simulink model "lab1_model"  (R2018a)
settings: Solver=VariableStepAuto  StartTime=0.0  StopTime=8  RelTol=1e-3
values from neighbouring files (symbols this model uses):
  Jtot = 7.226    [Lab1_script.m]
  Kb = 2    [Lab1_script.m]
  KCS = 0.5    [Lab1_script.m]
  Kf = 0.1    [Lab1_script.m]
  KSS = 0.0433    [Lab1_script.m]
  ntotKt = 1.8    [Lab1_script.m]
  r_itot = 0.0615    [Lab1_script.m]
  Ra = 1    [Lab1_script.m]
  RocwAvor_itot = 0.6154    [Lab1_script.m]
libraries: simulink x3
settings Model: Creator=Mohamed Badr  LastModifiedBy=Mohamed Badr

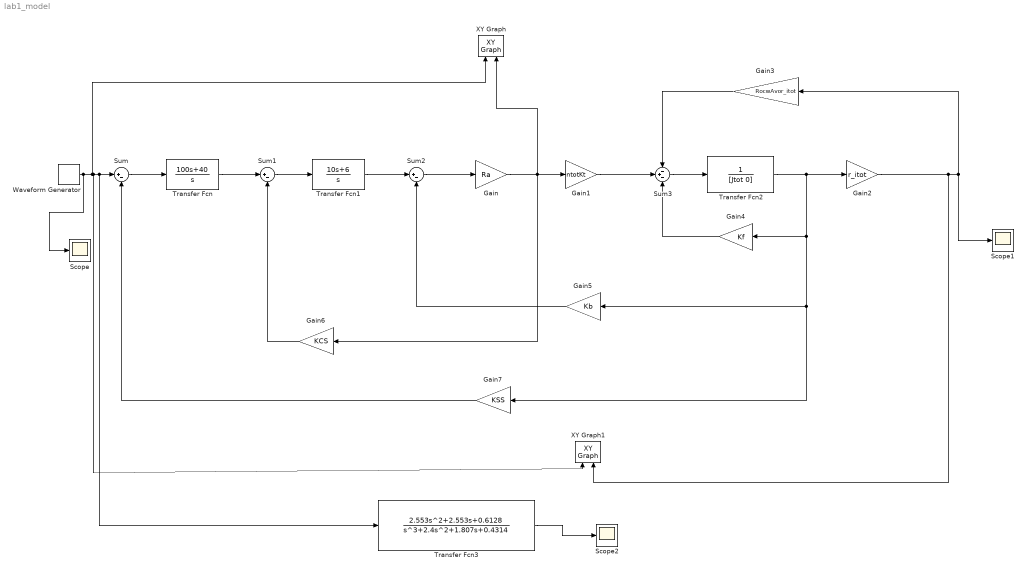
== system lab1_model ==
  Gain : Gain  Gain=Ra
  Gain1 : Gain  Gain=ntotKt
  Gain2 : Gain  Gain=r_itot
  Gain3 : Gain  Gain=RocwAvor_itot
  Gain4 : Gain  Gain=Kf
  Gain5 : Gain  Gain=Kb
  Gain6 : Gain  Gain=KCS
  Gain7 : Gain  Gain=KSS
  Scope : Scope
  Scope1 : Scope
  Scope2 : Scope
  Sum : Sum  Inputs=|+-
  Sum1 : Sum  Inputs=|+-
  Sum2 : Sum  Inputs=|+-
  Sum3 : Sum  Inputs=-+-
  Transfer Fcn : TransferFcn  Numerator=[100 40]  Denominator=[1 0]
  Transfer Fcn1 : TransferFcn  Numerator=[10 6]  Denominator=[1 0]
  Transfer Fcn2 : TransferFcn  Numerator=[0 1]  Denominator=[Jtot 0]
  Transfer Fcn3 : TransferFcn  Numerator=[0 2.553 2.553 0.6128]  Denominator=[1 2.4 1.807 0.4314]
  Waveform Generator : simulink/Sources/Waveform Generator  OutMin=[]  OutMax=[]  OutDataTypeStr=double  SelectedSignal=1  Signals=sawtooth('Amplitude',2.5,'Frequency',10)#step('StepTime',0,'InitialValue',0,'FinalValue',1)  BlockNames=MultiportSwitch_79321b648dd0437#MultiportSwitch_d5c94f2860884f4  SampleTime=0.1
      settings: SourceProductName=Simulink
  XY Graph : simulink/Sinks/XY Graph  xmin=-5  xmax=5  ymin=-5  ymax=10  st=-1
  XY Graph1 : simulink/Sinks/XY Graph  xmin=-5  xmax=5  ymin=-5  ymax=5  st=-1
  wires:
  Waveform Generator/1 -> Scope/1, XY Graph/1, XY Graph1/1, Transfer Fcn3/1, Sum/1
  Sum/1 -> Transfer Fcn/1
  Transfer Fcn/1 -> Sum1/1
  Sum1/1 -> Transfer Fcn1/1
  Transfer Fcn1/1 -> Sum2/1
  Sum2/1 -> Gain/1
  Gain/1 -> Gain6/1, XY Graph/2, Gain1/1
  Sum3/1 -> Transfer Fcn2/1
  Transfer Fcn2/1 -> Gain7/1, Gain5/1, Gain4/1, Gain2/1
  Gain3/1 -> Sum3/1
  Gain4/1 -> Sum3/3
  Gain1/1 -> Sum3/2
  Gain5/1 -> Sum2/2
  Gain6/1 -> Sum1/2
  Gain7/1 -> Sum/2
  Gain2/1 -> XY Graph1/2, Scope1/1, Gain3/1
  Transfer Fcn3/1 -> Scope2/1
